simulink model "kranTest"  (R2018b)
settings: Solver=VariableStepAuto  StartTime=0.0  StopTime=Tsim  FixedStep=0.005  RelTol=1e-4
model workspace: external: MATLAB File kran_DataFile.m (data not in the file)
values from neighbouring files (symbols this model uses):
  refPointsVector = [pointThree, pointOne, pointThree, pointTwo, pointThree]    [simulate_driving.m]    (also in testDriving.m)
  Ts = 50e-3    (= 0.05)    [simulation_params.m]    (also in testDriving.m = 0.1)
undefined symbols (not defined in the file or in its folder): EvaluateTrajectory, smiData, X, Y, Z
libraries: sm_lib x105, nesl_utility x32, fl_lib x27, sh_lib x9, elec_lib x2
(part 1 of 4)
settings Model: Creator=Marko  LastModifiedBy=Marko
settings SimscapeCC: SimscapeLogType=all  SimscapeLogSimulationStatistics=on  SimscapeLogLimitData=off
settings ExplorerConfigSet: InternalSimMechanicsExplorerSettings="<ExplorerConfiguration><canonicalview>planar_xy</canonicalview><AnimationSetting><BasePlaybackSpeed>1.0</BasePlaybackSpeed><PlaybackSpeedFactor>1.0</PlaybackSpeedFactor></AnimationSetting><TilePanel><TileInfo><Tiles Columns=\"1\" Count=\"1\" Rows=\"1\"><Column Weight=\"1\"/><Row Weight=\"1\"/><Tile Height=\"1\" Width=\"1\" X=\"0\" Y=\"0\"/></Tiles></TileInfo><SceneInfo><SceneViewer><BGColor><R>0.60000002384185791</R><G>0.60000002384185791</G><B>0.60000002384185791</B></BGColor><Camera><DoPerspective>off</DoPerspective><Position><X>10.1383469879859511</X><Y>3.51643315137439361</Y><Z>-1.36564695488922516</Z></Position><Center><X>1.28157942243814538</X><Y>3.51643315137439361</Y><Z>-1.36564695488922516</Z></Center><Up><X>0</X><Y>1</Y><Z>0</Z></Up><ViewLimDist>1</ViewLimDist><YLim>6.81084416950491534</YLim><XLim>4.8510498406429976</XLim></Camera></SceneViewer></SceneInfo></TilePanel><MechEditorPanel><Cameras/><GfxPanelCameraMap/><VideoCreator><PlaybackSpeedRatio>1.0</PlaybackSpeedRatio><FrameRate>30</FrameRate><VideoFormat>Motion JPEG AVI</VideoFormat><FrameSize>auto</FrameSize></VideoCreator></MechEditorPanel></ExplorerConfiguration>"

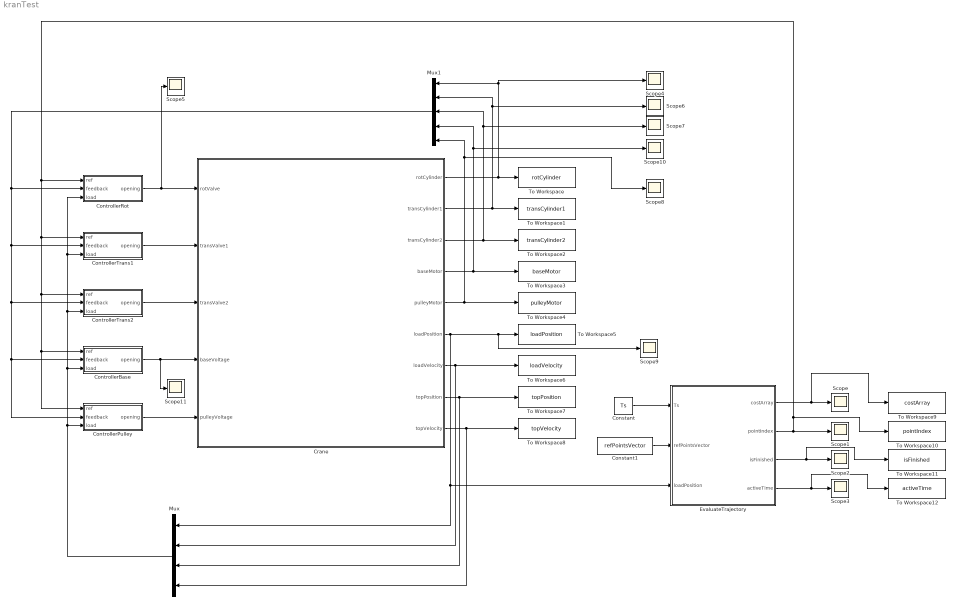
== system kranTest ==
  Constant : Constant  Value=Ts  SampleTime=-1
  Constant1 : Constant  Value=refPointsVector  SampleTime=-1
  ControllerBase : Subsystem
  ControllerPulley : Subsystem
  ControllerRot : Subsystem
  ControllerTrans1 : Subsystem
  ControllerTrans2 : Subsystem
  Crane : Subsystem
  EvaluateTrajectory : Subsystem
  Mux : Mux
  Mux1 : Mux  Inputs=5
  Scope{,1..11} (12 alike) : Scope
  To Workspace : ToWorkspace  VariableName=rotCylinder  SaveFormat=Structure With Time  SampleTime=Ts
  To Workspace1 : ToWorkspace  VariableName=transCylinder1  SaveFormat=Structure With Time  SampleTime=Ts
  To Workspace10 : ToWorkspace  VariableName=pointIndex  SaveFormat=Structure With Time  SampleTime=Ts
  To Workspace11 : ToWorkspace  VariableName=isFinished  SaveFormat=Structure With Time  SampleTime=Ts
  To Workspace12 : ToWorkspace  VariableName=activeTime  SaveFormat=Structure With Time  SampleTime=Ts
  To Workspace2 : ToWorkspace  VariableName=transCylinder2  SaveFormat=Structure With Time  SampleTime=Ts
  To Workspace3 : ToWorkspace  VariableName=baseMotor  SaveFormat=Structure With Time  SampleTime=Ts
  To Workspace4 : ToWorkspace  VariableName=pulleyMotor  SaveFormat=Structure With Time  SampleTime=Ts
  To Workspace5 : ToWorkspace  VariableName=loadPosition  SaveFormat=Structure With Time  SampleTime=Ts
  To Workspace6 : ToWorkspace  VariableName=loadVelocity  SaveFormat=Structure With Time  SampleTime=Ts
  To Workspace7 : ToWorkspace  VariableName=topPosition  SaveFormat=Structure With Time  SampleTime=Ts
  To Workspace8 : ToWorkspace  VariableName=topVelocity  SaveFormat=Structure With Time  SampleTime=Ts
  To Workspace9 : ToWorkspace  VariableName=costArray  SaveFormat=Structure With Time  SampleTime=Ts
  wires:
  Crane/1(rotCylinder) -> Scope4/1, Mux1/1, To Workspace/1
  Crane/2(transCylinder1) -> Mux1/2, Scope6/1, To Workspace1/1
  Crane/3(transCylinder2) -> Scope7/1, Mux1/3, To Workspace2/1
  Crane/4(baseMotor) -> Scope10/1, Mux1/4, To Workspace3/1
  Crane/5(pulleyMotor) -> Mux1/5, Scope8/1, To Workspace4/1
  Crane/6(loadPosition) -> Scope9/1, To Workspace5/1, EvaluateTrajectory/3(loadPosition), Mux/1
  Crane/7(loadVelocity) -> Mux/2, To Workspace6/1
  Crane/8(topPosition) -> Mux/3, To Workspace7/1
  Crane/9(topVelocity) -> Mux/4, To Workspace8/1
  Mux/1 -> ControllerRot/3(load), ControllerTrans1/3(load), ControllerTrans2/3(load), ControllerBase/3(load), ControllerPulley/3(load)
  Constant/1 -> EvaluateTrajectory/1(Ts)
  Constant1/1 -> EvaluateTrajectory/2(refPointsVector)
  EvaluateTrajectory/1(costArray) -> To Workspace9/1, Scope/1
  EvaluateTrajectory/3(isFinished) -> To Workspace11/1, Scope2/1
  EvaluateTrajectory/4(activeTime) -> To Workspace12/1, Scope3/1
  EvaluateTrajectory/2(pointIndex) -> To Workspace10/1, ControllerRot/1(ref), ControllerPulley/1(ref), ControllerBase/1(ref), ControllerTrans2/1(ref), ControllerTrans1/1(ref), Scope1/1
  Mux1/1 -> ControllerRot/2(feedback), ControllerTrans1/2(feedback), ControllerTrans2/2(feedback), ControllerPulley/2(feedback), ControllerBase/2(feedback)
  ControllerRot/1(opening) -> Scope5/1, Crane/1(rotValve)
  ControllerTrans1/1(opening) -> Crane/2(transValve1)
  ControllerTrans2/1(opening) -> Crane/3(transValve2)
  ControllerPulley/1(opening) -> Crane/5(pulleyVoltage)
  ControllerBase/1(opening) -> Scope11/1, Crane/4(baseVoltage)

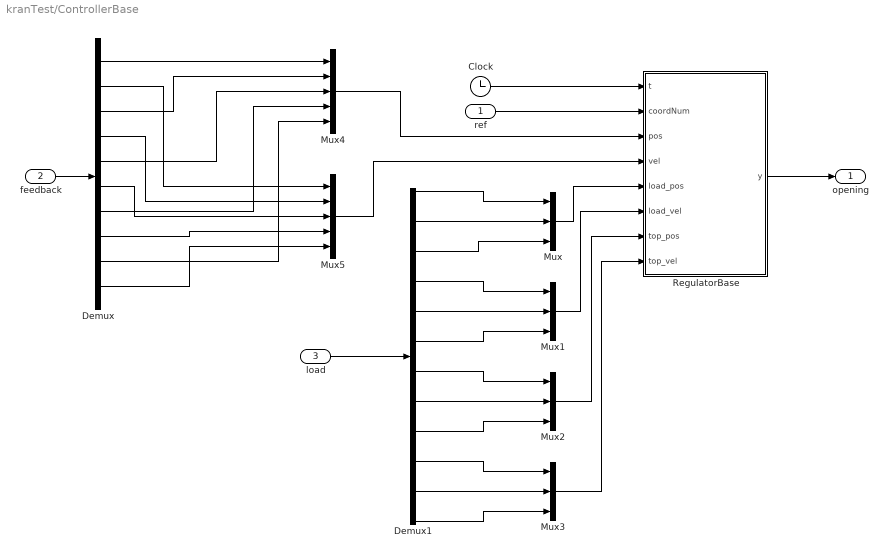
== system kranTest/ControllerBase ==
  ref : Inport
  feedback : Inport  Port=2
  load : Inport  Port=3
  Clock : Clock
  Demux : Demux  Outputs=10
  Demux1 : Demux  Outputs=12
  Mux{,1..3} (4 alike) : Mux  Inputs=3
  Mux4 : Mux  Inputs=5
  Mux5 : Mux  Inputs=5
  RegulatorBase : MATLAB Function  TreatAsAtomicUnit=on  SystemSampleTime=Ts
  opening : Outport
  wires:
  Demux1/7 -> Mux2/1
  Clock/1 -> RegulatorBase/1(t)
  Demux1/2 -> Mux/2
  Demux1/8 -> Mux2/2
  Mux1/1 -> RegulatorBase/6(load_vel)
  load/1 -> Demux1/1
  Demux1/1 -> Mux/1
  Demux1/10 -> Mux3/1
  Mux/1 -> RegulatorBase/5(load_pos)
  Mux3/1 -> RegulatorBase/8(top_vel)
  Demux1/6 -> Mux1/3
  Demux1/9 -> Mux2/3
  Mux2/1 -> RegulatorBase/7(top_pos)
  Demux1/5 -> Mux1/2
  Demux1/3 -> Mux/3
  Demux1/11 -> Mux3/2
  ref/1 -> RegulatorBase/2(coordNum)
  Demux1/12 -> Mux3/3
  RegulatorBase/1(y) -> opening/1
  Demux1/4 -> Mux1/1
  Mux4/1 -> RegulatorBase/3(pos)
  Demux/6 -> Mux5/3
  Demux/4 -> Mux5/2
  Demux/8 -> Mux5/4
  Demux/10 -> Mux5/5
  Demux/2 -> Mux5/1
  Demux/5 -> Mux4/3
  Demux/9 -> Mux4/5
  Demux/3 -> Mux4/2
  Demux/1 -> Mux4/1
  Demux/7 -> Mux4/4
  feedback/1 -> Demux/1
  Mux5/1 -> RegulatorBase/4(vel)

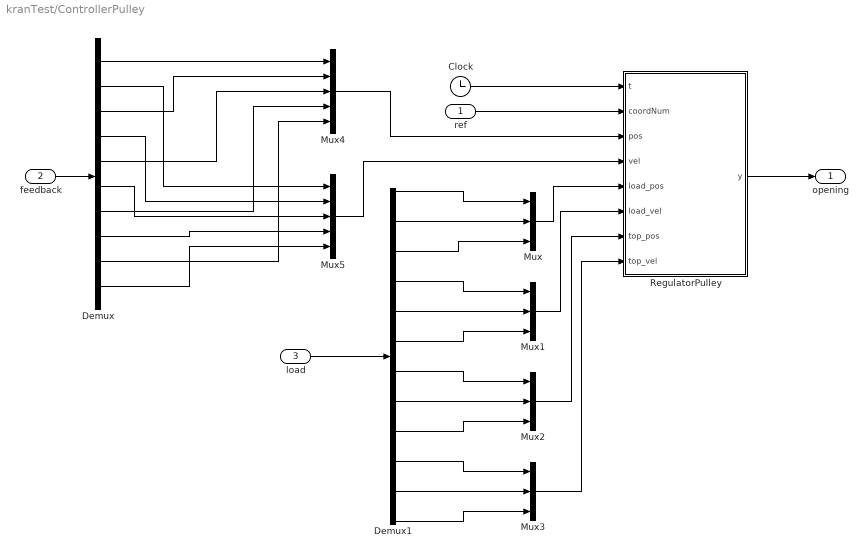
== system kranTest/ControllerPulley ==
  ref : Inport
  feedback : Inport  Port=2
  load : Inport  Port=3
  Clock : Clock
  Demux : Demux  Outputs=10
  Demux1 : Demux  Outputs=12
  Mux{,1..3} (4 alike) : Mux  Inputs=3
  Mux4 : Mux  Inputs=5
  Mux5 : Mux  Inputs=5
  RegulatorPulley : MATLAB Function  TreatAsAtomicUnit=on  SystemSampleTime=Ts
  opening : Outport
  wires:
  Demux1/7 -> Mux2/1
  Clock/1 -> RegulatorPulley/1(t)
  Demux1/2 -> Mux/2
  Demux1/8 -> Mux2/2
  Mux1/1 -> RegulatorPulley/6(load_vel)
  load/1 -> Demux1/1
  Demux1/1 -> Mux/1
  Demux1/10 -> Mux3/1
  Mux/1 -> RegulatorPulley/5(load_pos)
  Mux3/1 -> RegulatorPulley/8(top_vel)
  Demux1/6 -> Mux1/3
  Demux1/9 -> Mux2/3
  Mux2/1 -> RegulatorPulley/7(top_pos)
  Demux1/5 -> Mux1/2
  Demux1/3 -> Mux/3
  Demux1/11 -> Mux3/2
  ref/1 -> RegulatorPulley/2(coordNum)
  Demux1/12 -> Mux3/3
  RegulatorPulley/1(y) -> opening/1
  Demux1/4 -> Mux1/1
  Demux/6 -> Mux5/3
  Demux/4 -> Mux5/2
  Demux/8 -> Mux5/4
  Demux/10 -> Mux5/5
  Demux/2 -> Mux5/1
  Demux/5 -> Mux4/3
  Demux/9 -> Mux4/5
  Demux/3 -> Mux4/2
  Demux/1 -> Mux4/1
  Demux/7 -> Mux4/4
  feedback/1 -> Demux/1
  Mux4/1 -> RegulatorPulley/3(pos)
  Mux5/1 -> RegulatorPulley/4(vel)

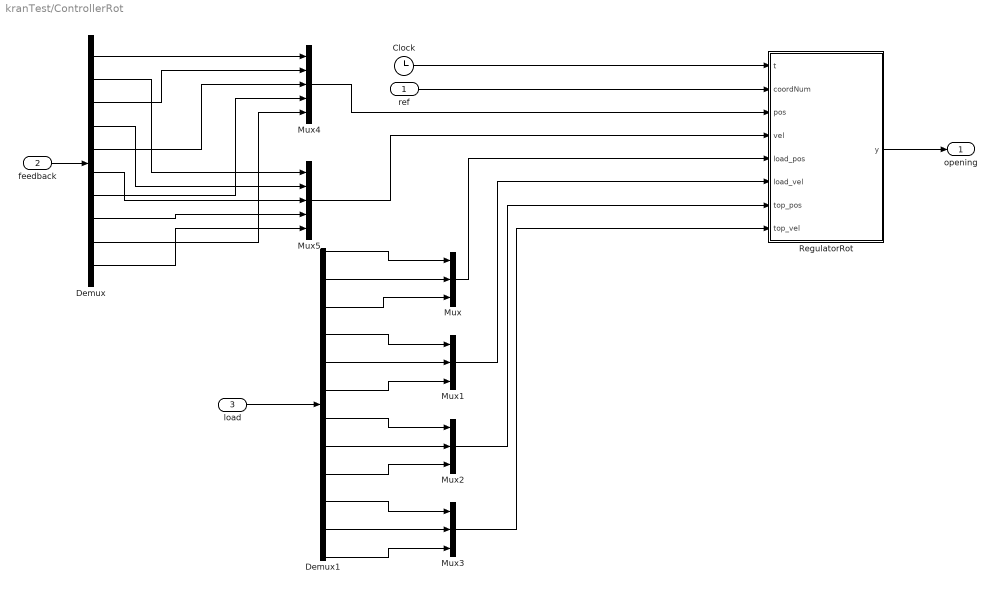
== system kranTest/ControllerRot ==
  ref : Inport
  feedback : Inport  Port=2
  load : Inport  Port=3
  Clock : Clock
  Demux : Demux  Outputs=10
  Demux1 : Demux  Outputs=12
  Mux{,1..3} (4 alike) : Mux  Inputs=3
  Mux4 : Mux  Inputs=5
  Mux5 : Mux  Inputs=5
  RegulatorRot : MATLAB Function  TreatAsAtomicUnit=on  SystemSampleTime=Ts
  opening : Outport
  wires:
  RegulatorRot/1(y) -> opening/1
  ref/1 -> RegulatorRot/2(coordNum)
  Clock/1 -> RegulatorRot/1(t)
  load/1 -> Demux1/1
  Mux/1 -> RegulatorRot/5(load_pos)
  Mux1/1 -> RegulatorRot/6(load_vel)
  Mux2/1 -> RegulatorRot/7(top_pos)
  Mux3/1 -> RegulatorRot/8(top_vel)
  Demux1/1 -> Mux/1
  Demux1/2 -> Mux/2
  Demux1/3 -> Mux/3
  Demux1/4 -> Mux1/1
  Demux1/5 -> Mux1/2
  Demux1/6 -> Mux1/3
  Demux1/7 -> Mux2/1
  Demux1/8 -> Mux2/2
  Demux1/9 -> Mux2/3
  Demux1/10 -> Mux3/1
  Demux1/11 -> Mux3/2
  Demux1/12 -> Mux3/3
  Demux/1 -> Mux4/1
  Demux/3 -> Mux4/2
  Demux/5 -> Mux4/3
  Demux/7 -> Mux4/4
  Demux/9 -> Mux4/5
  Demux/2 -> Mux5/1
  Demux/4 -> Mux5/2
  Demux/6 -> Mux5/3
  Demux/8 -> Mux5/4
  Demux/10 -> Mux5/5
  Mux4/1 -> RegulatorRot/3(pos)
  Mux5/1 -> RegulatorRot/4(vel)
  feedback/1 -> Demux/1

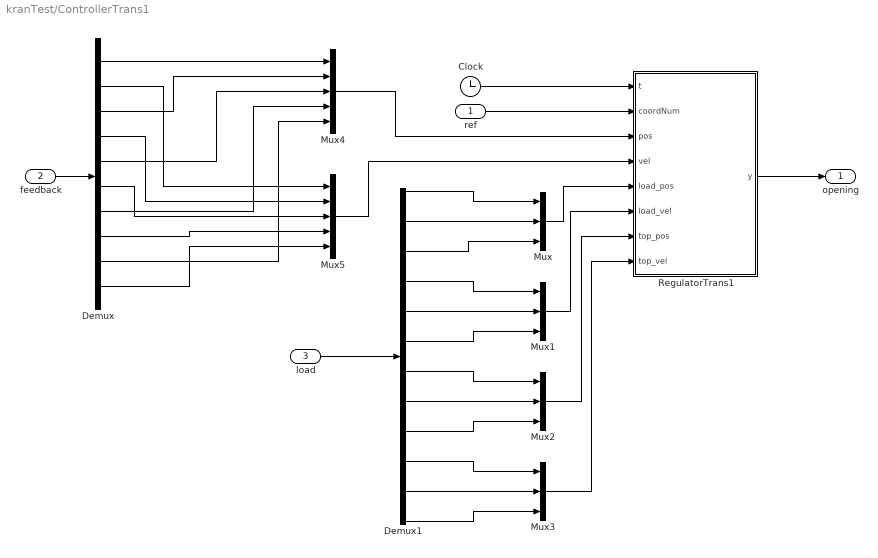
== system kranTest/ControllerTrans1 ==
  ref : Inport
  feedback : Inport  Port=2
  load : Inport  Port=3
  Clock : Clock
  Demux : Demux  Outputs=10
  Demux1 : Demux  Outputs=12
  Mux{,1..3} (4 alike) : Mux  Inputs=3
  Mux4 : Mux  Inputs=5
  Mux5 : Mux  Inputs=5
  RegulatorTrans1 : MATLAB Function  TreatAsAtomicUnit=on  SystemSampleTime=Ts
  opening : Outport
  wires:
  Demux1/7 -> Mux2/1
  Clock/1 -> RegulatorTrans1/1(t)
  Demux1/2 -> Mux/2
  Demux1/8 -> Mux2/2
  Mux1/1 -> RegulatorTrans1/6(load_vel)
  load/1 -> Demux1/1
  Demux1/1 -> Mux/1
  Demux1/10 -> Mux3/1
  Mux/1 -> RegulatorTrans1/5(load_pos)
  Mux3/1 -> RegulatorTrans1/8(top_vel)
  Demux1/6 -> Mux1/3
  Demux1/9 -> Mux2/3
  Mux2/1 -> RegulatorTrans1/7(top_pos)
  Demux1/5 -> Mux1/2
  Demux1/3 -> Mux/3
  Demux1/11 -> Mux3/2
  ref/1 -> RegulatorTrans1/2(coordNum)
  Demux1/12 -> Mux3/3
  RegulatorTrans1/1(y) -> opening/1
  Demux1/4 -> Mux1/1
  Demux/6 -> Mux5/3
  Demux/4 -> Mux5/2
  Demux/8 -> Mux5/4
  Demux/10 -> Mux5/5
  Demux/2 -> Mux5/1
  Demux/5 -> Mux4/3
  Demux/9 -> Mux4/5
  Demux/3 -> Mux4/2
  Demux/1 -> Mux4/1
  Demux/7 -> Mux4/4
  feedback/1 -> Demux/1
  Mux4/1 -> RegulatorTrans1/3(pos)
  Mux5/1 -> RegulatorTrans1/4(vel)

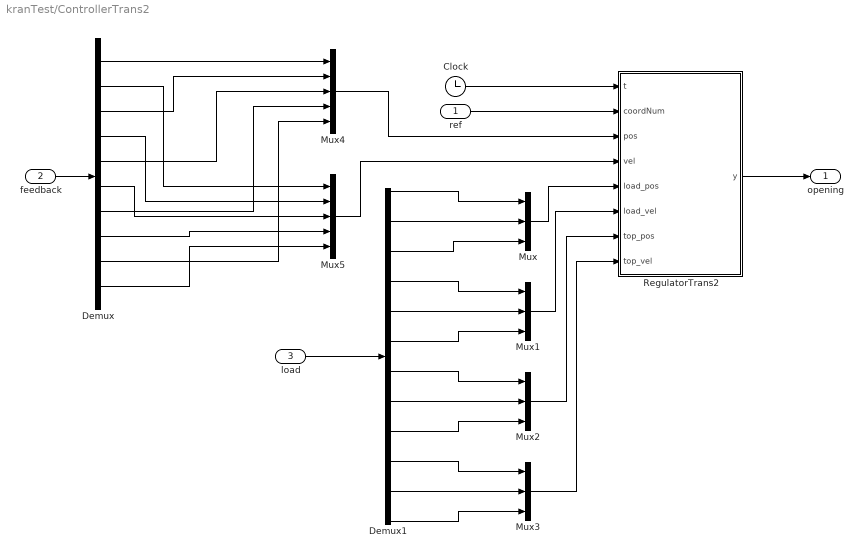
== system kranTest/ControllerTrans2 ==
  ref : Inport
  feedback : Inport  Port=2
  load : Inport  Port=3
  Clock : Clock
  Demux : Demux  Outputs=10
  Demux1 : Demux  Outputs=12
  Mux{,1..3} (4 alike) : Mux  Inputs=3
  Mux4 : Mux  Inputs=5
  Mux5 : Mux  Inputs=5
  RegulatorTrans2 : MATLAB Function  TreatAsAtomicUnit=on  SystemSampleTime=Ts
  opening : Outport
  wires:
  Demux1/7 -> Mux2/1
  Clock/1 -> RegulatorTrans2/1(t)
  Demux1/2 -> Mux/2
  Demux1/8 -> Mux2/2
  Mux1/1 -> RegulatorTrans2/6(load_vel)
  load/1 -> Demux1/1
  Demux1/1 -> Mux/1
  Demux1/10 -> Mux3/1
  Mux/1 -> RegulatorTrans2/5(load_pos)
  Mux3/1 -> RegulatorTrans2/8(top_vel)
  Demux1/6 -> Mux1/3
  Demux1/9 -> Mux2/3
  Mux2/1 -> RegulatorTrans2/7(top_pos)
  Demux1/5 -> Mux1/2
  Demux1/3 -> Mux/3
  Demux1/11 -> Mux3/2
  ref/1 -> RegulatorTrans2/2(coordNum)
  Demux1/12 -> Mux3/3
  RegulatorTrans2/1(y) -> opening/1
  Demux1/4 -> Mux1/1
  Demux/6 -> Mux5/3
  Demux/4 -> Mux5/2
  Demux/8 -> Mux5/4
  Demux/10 -> Mux5/5
  Demux/2 -> Mux5/1
  Demux/5 -> Mux4/3
  Demux/9 -> Mux4/5
  Demux/3 -> Mux4/2
  Demux/1 -> Mux4/1
  Demux/7 -> Mux4/4
  feedback/1 -> Demux/1
  Mux4/1 -> RegulatorTrans2/3(pos)
  Mux5/1 -> RegulatorTrans2/4(vel)

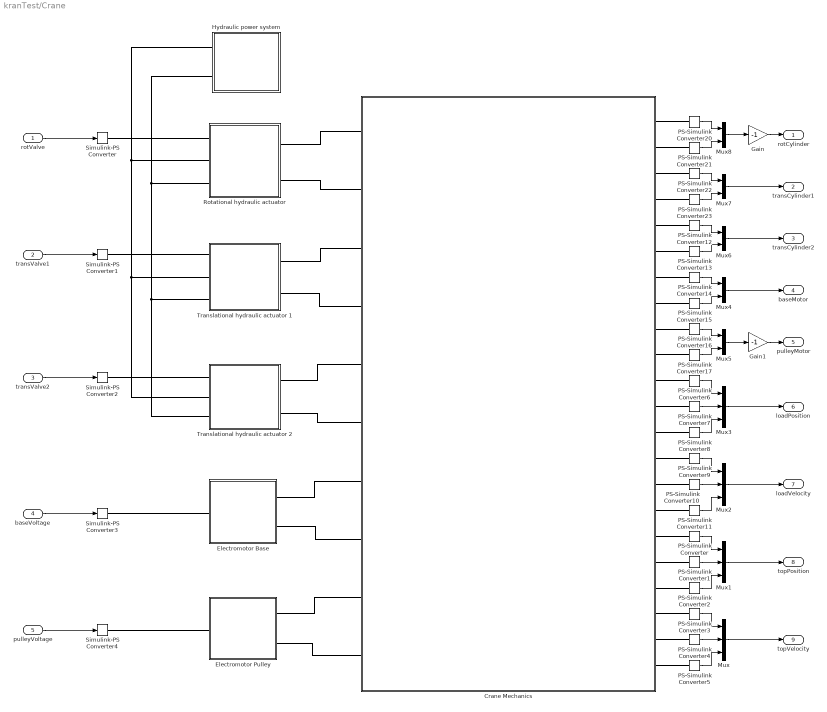
== system kranTest/Crane ==
  rotValve : Inport
  transValve1 : Inport  Port=2
  transValve2 : Inport  Port=3
  baseVoltage : Inport  Port=4
  pulleyVoltage : Inport  Port=5
  Crane Mechanics : Subsystem
  Electromotor Base : Subsystem
  Electromotor Pulley : Subsystem
  Gain : Gain  Gain=-1
  Gain1 : Gain  Gain=-1
  Hydraulic power system : Subsystem
  Mux{,1..3} (4 alike) : Mux  Inputs=3
  Mux{4..8} (5 alike) : Mux  Inputs=2
  PS-Simulink Converter{,1..17,20..23} (22 alike) : nesl_utility/PS-Simulink Converter  PhysicalDomain=network_engine_domain  SubClassName=ps_output  LeftPortType=input  RightPortType=output  PseudoPeriodic=off  Frequencies=[]  Unit=1  AffineConversion=off
  Rotational hydraulic actuator : Subsystem
  Simulink-PS Converter : nesl_utility/Simulink-PS Converter  PhysicalDomain=network_engine_domain  SubClassName=ps_input  LeftPortType=input  RightPortType=output  PseudoPeriodic=off  Frequencies=[]  NoiseDistribution=none  NoiseParameters=[]  Unit=1  AffineConversion=off  FilteringAndDerivatives=provide  SimscapeFilterOrder=1  InputFilterTimeConstant=0.001  UdotUserProvided=0
  Simulink-PS Converter{1..4} (4 alike) : nesl_utility/Simulink-PS Converter  PhysicalDomain=network_engine_domain  SubClassName=ps_input  LeftPortType=input  RightPortType=output  PseudoPeriodic=off  Frequencies=[]  NoiseDistribution=none  NoiseParameters=[]  Unit=1  AffineConversion=off  FilteringAndDerivatives=provide  SimscapeFilterOrder=2  InputFilterTimeConstant=0.001  UdotUserProvided=0
  Translational hydraulic actuator 1 : Subsystem
  Translational hydraulic actuator 2 : Subsystem
  rotCylinder : Outport
  transCylinder1 : Outport  Port=2
  transCylinder2 : Outport  Port=3
  baseMotor : Outport  Port=4
  pulleyMotor : Outport  Port=5
  loadPosition : Outport  Port=6
  loadVelocity : Outport  Port=7
  topPosition : Outport  Port=8
  topVelocity : Outport  Port=9
  wires:
  PS-Simulink Converter12/1 -> Mux6/1
  Mux2/1 -> loadVelocity/1
  PS-Simulink Converter11/1 -> Mux2/3
  PS-Simulink Converter22/1 -> Mux7/1
  Mux3/1 -> loadPosition/1
  PS-Simulink Converter4/1 -> Mux/2
  PS-Simulink Converter17/1 -> Mux5/2
  PS-Simulink Converter15/1 -> Mux4/2
  PS-Simulink Converter1/1 -> Mux1/2
  PS-Simulink Converter/1 -> Mux1/1
  PS-Simulink Converter21/1 -> Mux8/2
  PS-Simulink Converter9/1 -> Mux2/1
  PS-Simulink Converter8/1 -> Mux3/3
  PS-Simulink Converter10/1 -> Mux2/2
  PS-Simulink Converter6/1 -> Mux3/1
  PS-Simulink Converter14/1 -> Mux4/1
  PS-Simulink Converter13/1 -> Mux6/2
  Mux6/1 -> transCylinder2/1
  PS-Simulink Converter16/1 -> Mux5/1
  PS-Simulink Converter3/1 -> Mux/1
  PS-Simulink Converter20/1 -> Mux8/1
  PS-Simulink Converter23/1 -> Mux7/2
  Mux1/1 -> topPosition/1
  PS-Simulink Converter5/1 -> Mux/3
  PS-Simulink Converter2/1 -> Mux1/3
  PS-Simulink Converter7/1 -> Mux3/2
  Mux7/1 -> transCylinder1/1
  Mux4/1 -> baseMotor/1
  Mux/1 -> topVelocity/1
  Mux5/1 -> Gain1/1
  Mux8/1 -> Gain/1
  pulleyVoltage/1 -> Simulink-PS Converter4/1
  transValve1/1 -> Simulink-PS Converter1/1
  baseVoltage/1 -> Simulink-PS Converter3/1
  rotValve/1 -> Simulink-PS Converter/1
  transValve2/1 -> Simulink-PS Converter2/1
  Gain/1 -> rotCylinder/1
  Gain1/1 -> pulleyMotor/1
  connections:
  Crane Mechanics/RConn5 -- PS-Simulink Converter12/LConn1
  Hydraulic power system/RConn2 -- Rotational hydraulic actuator/LConn3 -- Translational hydraulic actuator 2/LConn3 -- Translational hydraulic actuator 1/LConn3
  Rotational hydraulic actuator/RConn2 -- Crane Mechanics/LConn2
  Crane Mechanics/RConn7 -- PS-Simulink Converter14/LConn1
  Hydraulic power system/RConn1 -- Rotational hydraulic actuator/LConn2 -- Translational hydraulic actuator 2/LConn2 -- Translational hydraulic actuator 1/LConn2
  Translational hydraulic actuator 1/RConn1 -- Crane Mechanics/LConn3
  Crane Mechanics/RConn14 -- PS-Simulink Converter9/LConn1
  Crane Mechanics/RConn6 -- PS-Simulink Converter13/LConn1
  Crane Mechanics/RConn15 -- PS-Simulink Converter10/LConn1
  Translational hydraulic actuator 2/RConn2 -- Crane Mechanics/LConn6
  Crane Mechanics/RConn9 -- PS-Simulink Converter16/LConn1
  Simulink-PS Converter4/RConn1 -- Electromotor Pulley/LConn1
  Electromotor Pulley/RConn2 -- Crane Mechanics/LConn10
  PS-Simulink Converter2/LConn1 -- Crane Mechanics/RConn19
  Crane Mechanics/RConn16 -- PS-Simulink Converter11/LConn1
  Crane Mechanics/RConn11 -- PS-Simulink Converter6/LConn1
  PS-Simulink Converter5/LConn1 -- Crane Mechanics/RConn22
  Rotational hydraulic actuator/RConn1 -- Crane Mechanics/LConn1
  Crane Mechanics/RConn4 -- PS-Simulink Converter23/LConn1
  Crane Mechanics/RConn13 -- PS-Simulink Converter8/LConn1
  Electromotor Base/RConn2 -- Crane Mechanics/LConn8
  Translational hydraulic actuator 1/RConn2 -- Crane Mechanics/LConn4
  PS-Simulink Converter/LConn1 -- Crane Mechanics/RConn17
  Crane Mechanics/RConn3 -- PS-Simulink Converter22/LConn1
  Crane Mechanics/LConn9 -- Electromotor Pulley/RConn1
  Crane Mechanics/RConn8 -- PS-Simulink Converter15/LConn1
  PS-Simulink Converter4/LConn1 -- Crane Mechanics/RConn21
  Crane Mechanics/RConn2 -- PS-Simulink Converter21/LConn1
  Crane Mechanics/LConn5 -- Translational hydraulic actuator 2/RConn1
  Simulink-PS Converter/RConn1 -- Rotational hydraulic actuator/LConn1
  Simulink-PS Converter3/RConn1 -- Electromotor Base/LConn1
  Simulink-PS Converter1/RConn1 -- Translational hydraulic actuator 1/LConn1
  Crane Mechanics/RConn12 -- PS-Simulink Converter7/LConn1
  Crane Mechanics/RConn1 -- PS-Simulink Converter20/LConn1
  Simulink-PS Converter2/RConn1 -- Translational hydraulic actuator 2/LConn1
  PS-Simulink Converter1/LConn1 -- Crane Mechanics/RConn18
  Crane Mechanics/LConn7 -- Electromotor Base/RConn1
  Crane Mechanics/RConn10 -- PS-Simulink Converter17/LConn1
  PS-Simulink Converter3/LConn1 -- Crane Mechanics/RConn20

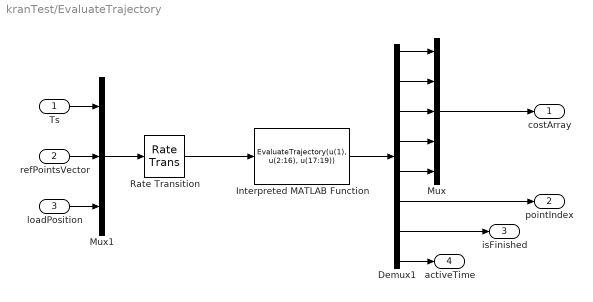
== system kranTest/EvaluateTrajectory ==
  Ts : Inport
  refPointsVector : Inport  Port=2
  loadPosition : Inport  Port=3
  Demux1 : Demux  Outputs=8
  Interpreted MATLAB Function : MATLABFcn  MATLABFcn=EvaluateTrajectory(u(1), u(2:16), u(17:19))  OutputDimensions=8  OutputSignalType=real
  Mux : Mux  Inputs=5
  Mux1 : Mux  Inputs=3
  Rate Transition : RateTransition  OutPortSampleTime=Ts
  costArray : Outport
  pointIndex : Outport  Port=2
  isFinished : Outport  Port=3
  activeTime : Outport  Port=4
  wires:
  Interpreted MATLAB Function/1 -> Demux1/1
  Rate Transition/1 -> Interpreted MATLAB Function/1
  Mux1/1 -> Rate Transition/1
  refPointsVector/1 -> Mux1/2
  Ts/1 -> Mux1/1
  loadPosition/1 -> Mux1/3
  Mux/1 -> costArray/1
  Demux1/1 -> Mux/1
  Demux1/2 -> Mux/2
  Demux1/3 -> Mux/3
  Demux1/4 -> Mux/4
  Demux1/5 -> Mux/5
  Demux1/6 -> pointIndex/1
  Demux1/7 -> isFinished/1
  Demux1/8 -> activeTime/1

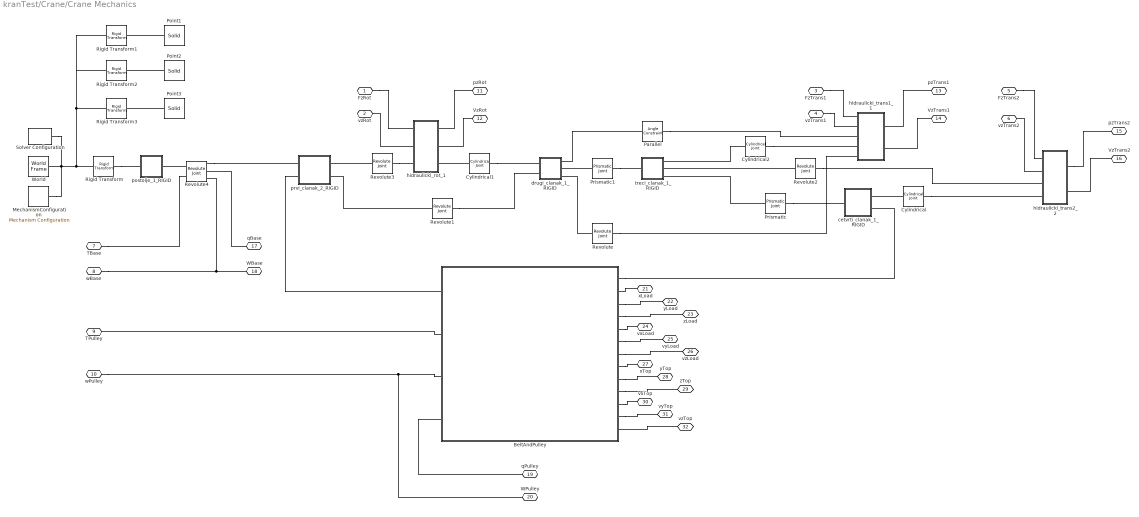
== system kranTest/Crane/Crane Mechanics ==
  BeltAndPulley : Subsystem
  Cylindrical : sm_lib/Joints/Cylindrical Joint  SenseConstraintForce=off  SenseConstraintForceX=off  SenseConstraintForceY=off  SenseConstraintForceZ=off  SenseConstraintTorque=off  SenseConstraintTorqueX=off  SenseConstraintTorqueY=off  SenseConstraintTorqueZ=off  SenseTotalForce=off  SenseTotalForceX=off  SenseTotalForceY=off  SenseTotalForceZ=off  SenseTotalTorque=off  SenseTotalTorqueX=off  SenseTotalTorqueY=off  SenseTotalTorqueZ=off  CompositeWrenchDir=FollowerOnBase  CompositeWrenchFrame=BaseFrame  PzEquilibriumPosition=0  PzEquilibriumPositionUnits=m  PzSpringStiffness=0  PzSpringStiffnessUnits=N/m  PzDampingCoefficient=0  PzDampingCoefficientUnits=N/(m/s)  PzTorqueActuationMode=NoTorque  PzMotionActuationMode=ComputedMotion  PzSensePosition=off  PzSenseVelocity=off  PzSenseAcceleration=off  PzSenseTorqueForce=off  PzPositionTargetSpecify=off  PzPositionTargetPriority=High  PzPositionTargetValue=0  PzPositionTargetValueUnits=m  PzVelocityTargetSpecify=off  PzVelocityTargetPriority=High  PzVelocityTargetValue=0  PzVelocityTargetValueUnits=m/s  RzEquilibriumPosition=0  RzEquilibriumPositionUnits=rad  RzSpringStiffness=0  RzSpringStiffnessUnits=N*m/rad  RzDampingCoefficient=0  RzDampingCoefficientUnits=N*m/(rad/s)  RzTorqueActuationMode=NoTorque  RzMotionActuationMode=ComputedMotion  RzSensePosition=off  RzSenseVelocity=off  RzSenseAcceleration=off  RzSenseTorqueForce=off  RzPositionTargetSpecify=off  RzPositionTargetPriority=High  RzPositionTargetValue=0  RzPositionTargetValueUnits=deg  RzVelocityTargetSpecify=off  RzVelocityTargetPriority=High  RzVelocityTargetValue=0  RzVelocityTargetValueUnits=deg/s
  Cylindrical1 : sm_lib/Joints/Cylindrical Joint  SenseConstraintForce=off  SenseConstraintForceX=off  SenseConstraintForceY=off  SenseConstraintForceZ=off  SenseConstraintTorque=off  SenseConstraintTorqueX=off  SenseConstraintTorqueY=off  SenseConstraintTorqueZ=off  SenseTotalForce=off  SenseTotalForceX=off  SenseTotalForceY=off  SenseTotalForceZ=off  SenseTotalTorque=off  SenseTotalTorqueX=off  SenseTotalTorqueY=off  SenseTotalTorqueZ=off  CompositeWrenchDir=FollowerOnBase  CompositeWrenchFrame=BaseFrame  PzEquilibriumPosition=0  PzEquilibriumPositionUnits=m  PzSpringStiffness=0  PzSpringStiffnessUnits=N/m  PzDampingCoefficient=0  PzDampingCoefficientUnits=N/(m/s)  PzTorqueActuationMode=NoTorque  PzMotionActuationMode=ComputedMotion  PzSensePosition=off  PzSenseVelocity=off  PzSenseAcceleration=off  PzSenseTorqueForce=off  PzPositionTargetSpecify=off  PzPositionTargetPriority=High  PzPositionTargetValue=0  PzPositionTargetValueUnits=m  PzVelocityTargetSpecify=off  PzVelocityTargetPriority=High  PzVelocityTargetValue=0  PzVelocityTargetValueUnits=m/s  RzEquilibriumPosition=0  RzEquilibriumPositionUnits=rad  RzSpringStiffness=0  RzSpringStiffnessUnits=N*m/rad  RzDampingCoefficient=0  RzDampingCoefficientUnits=N*m/(rad/s)  RzTorqueActuationMode=NoTorque  RzMotionActuationMode=ComputedMotion  RzSensePosition=off  RzSenseVelocity=off  RzSenseAcceleration=off  RzSenseTorqueForce=off  RzPositionTargetSpecify=off  RzPositionTargetPriority=High  RzPositionTargetValue=0  RzPositionTargetValueUnits=deg  RzVelocityTargetSpecify=off  RzVelocityTargetPriority=High  RzVelocityTargetValue=0  RzVelocityTargetValueUnits=deg/s
  Cylindrical2 : sm_lib/Joints/Cylindrical Joint  SenseConstraintForce=off  SenseConstraintForceX=off  SenseConstraintForceY=off  SenseConstraintForceZ=off  SenseConstraintTorque=off  SenseConstraintTorqueX=off  SenseConstraintTorqueY=off  SenseConstraintTorqueZ=off  SenseTotalForce=off  SenseTotalForceX=off  SenseTotalForceY=off  SenseTotalForceZ=off  SenseTotalTorque=off  SenseTotalTorqueX=off  SenseTotalTorqueY=off  SenseTotalTorqueZ=off  CompositeWrenchDir=FollowerOnBase  CompositeWrenchFrame=BaseFrame  PzEquilibriumPosition=0  PzEquilibriumPositionUnits=m  PzSpringStiffness=0  PzSpringStiffnessUnits=N/m  PzDampingCoefficient=0  PzDampingCoefficientUnits=N/(m/s)  PzTorqueActuationMode=NoTorque  PzMotionActuationMode=ComputedMotion  PzSensePosition=off  PzSenseVelocity=off  PzSenseAcceleration=off  PzSenseTorqueForce=off  PzPositionTargetSpecify=off  PzPositionTargetPriority=High  PzPositionTargetValue=0  PzPositionTargetValueUnits=m  PzVelocityTargetSpecify=off  PzVelocityTargetPriority=High  PzVelocityTargetValue=0  PzVelocityTargetValueUnits=m/s  RzEquilibriumPosition=0  RzEquilibriumPositionUnits=rad  RzSpringStiffness=0  RzSpringStiffnessUnits=N*m/rad  RzDampingCoefficient=0  RzDampingCoefficientUnits=N*m/(rad/s)  RzTorqueActuationMode=NoTorque  RzMotionActuationMode=ComputedMotion  RzSensePosition=off  RzSenseVelocity=off  RzSenseAcceleration=off  RzSenseTorqueForce=off  RzPositionTargetSpecify=off  RzPositionTargetPriority=High  RzPositionTargetValue=0  RzPositionTargetValueUnits=deg  RzVelocityTargetSpecify=off  RzVelocityTargetPriority=High  RzVelocityTargetValue=0  RzVelocityTargetValueUnits=deg/s
  MechanismConfiguration : sm_lib/Utilities/Mechanism Configuration  UniformGravity=Constant  GravityVector=[0 -9.80665 0]  GravityUnits=m/s^2  LinearizationDelta=0.001
  Parallel : sm_lib/Constraints/Angle Constraint  ConstraintType=Parallel  Angle=45  AngleUnits=deg  SenseSignedTorqueMagnitude=off  SenseTorque=off  SenseForce=off  WrenchDir=FollowerOnBase  WrenchFrame=BaseFrame
      settings: SourceProductName=Simscape Multibody  SourceProductBaseCode=MS
  Point1 : sm_lib/Body Elements/Solid  InertiaType=CalculateFromGeometry  Mass=1  MassUnits=kg  CenterOfMass=[0 0 0]  CenterOfMassUnits=m  MomentsOfInertia=[1 1 1]  MomentsOfInertiaUnits=kg*m^2  ProductsOfInertia=[0 0 0]  ProductsOfInertiaUnits=kg*m^2  BasedOnType=Density  Density=1000  DensityUnits=kg/m^3  DoExposeReferenceFrame=on  SerializedFrames=<Frames/>  GraphicType=FromGeometry  MarkerShape=Sphere  MarkerSize=10  GraphicVisPropType=AdvancedVisualProperties  GraphicDiffuseColor=[0 1 0]  GraphicSpecularColor=[0.5 0.5 0.5 1.0]  GraphicAmbientColor=[0.15 0.15 0.15 1.0]  GraphicEmissiveColor=[0.0 0.0 0.0 1.0]  GraphicShininess=75  GraphicOpacity=1.0  GeometryShape=Sphere  RectangleSize=[1 1]  RectangleSizeUnits=m  BrickDimensions=[1 1 1]  BrickDimensionUnits=m  CylinderRadius=1  CylinderRadiusUnits=m  CylinderLength=1  CylinderLengthUnits=m  SphereRadius=0.25  SphereRadiusUnits=m  EllipsoidRadii=[1 1 1]  EllipsoidRadiiUnits=m  ExtrusionCrossSection=[1 1; -1 1; -1 -1; 1 -1]  ExtrusionCrossSectionUnits=m  ExtrusionLength=1  ExtrusionLengthUnits=m  PolygonNumSides=3  PolygonOuterRadius=1  PolygonOuterRadiusUnits=m  ExtGeomFileType=STEP  ExtGeomFileUnits=m  RevolutionCrossSection=[1 1; 1 -1; 2 -1; 2 1]  RevolutionCrossSectionUnits=m  RevolutionExtent=Full  RevolutionAngle=180  RevolutionAngleUnits=deg
  Point2 : sm_lib/Body Elements/Solid  InertiaType=CalculateFromGeometry  Mass=1  MassUnits=kg  CenterOfMass=[0 0 0]  CenterOfMassUnits=m  MomentsOfInertia=[1 1 1]  MomentsOfInertiaUnits=kg*m^2  ProductsOfInertia=[0 0 0]  ProductsOfInertiaUnits=kg*m^2  BasedOnType=Density  Density=1000  DensityUnits=kg/m^3  DoExposeReferenceFrame=on  SerializedFrames=<Frames/>  GraphicType=FromGeometry  MarkerShape=Sphere  MarkerSize=10  GraphicVisPropType=AdvancedVisualProperties  GraphicDiffuseColor=[0 0 1]  GraphicSpecularColor=[0.5 0.5 0.5 1.0]  GraphicAmbientColor=[0.15 0.15 0.15 1.0]  GraphicEmissiveColor=[0.0 0.0 0.0 1.0]  GraphicShininess=75  GraphicOpacity=1.0  GeometryShape=Sphere  RectangleSize=[1 1]  RectangleSizeUnits=m  BrickDimensions=[1 1 1]  BrickDimensionUnits=m  CylinderRadius=1  CylinderRadiusUnits=m  CylinderLength=1  CylinderLengthUnits=m  SphereRadius=0.25  SphereRadiusUnits=m  EllipsoidRadii=[1 1 1]  EllipsoidRadiiUnits=m  ExtrusionCrossSection=[1 1; -1 1; -1 -1; 1 -1]  ExtrusionCrossSectionUnits=m  ExtrusionLength=1  ExtrusionLengthUnits=m  PolygonNumSides=3  PolygonOuterRadius=1  PolygonOuterRadiusUnits=m  ExtGeomFileType=STEP  ExtGeomFileUnits=m  RevolutionCrossSection=[1 1; 1 -1; 2 -1; 2 1]  RevolutionCrossSectionUnits=m  RevolutionExtent=Full  RevolutionAngle=180  RevolutionAngleUnits=deg
  Point3 : sm_lib/Body Elements/Solid  InertiaType=CalculateFromGeometry  Mass=1  MassUnits=kg  CenterOfMass=[0 0 0]  CenterOfMassUnits=m  MomentsOfInertia=[1 1 1]  MomentsOfInertiaUnits=kg*m^2  ProductsOfInertia=[0 0 0]  ProductsOfInertiaUnits=kg*m^2  BasedOnType=Density  Density=1000  DensityUnits=kg/m^3  DoExposeReferenceFrame=on  SerializedFrames=<Frames/>  GraphicType=FromGeometry  MarkerShape=Sphere  MarkerSize=10  GraphicVisPropType=AdvancedVisualProperties  GraphicDiffuseColor=[1 0 0]  GraphicSpecularColor=[0.5 0.5 0.5 1.0]  GraphicAmbientColor=[0.15 0.15 0.15 1.0]  GraphicEmissiveColor=[0.0 0.0 0.0 1.0]  GraphicShininess=75  GraphicOpacity=1.0  GeometryShape=Sphere  RectangleSize=[1 1]  RectangleSizeUnits=m  BrickDimensions=[1 1 1]  BrickDimensionUnits=m  CylinderRadius=1  CylinderRadiusUnits=m  CylinderLength=1  CylinderLengthUnits=m  SphereRadius=0.25  SphereRadiusUnits=m  EllipsoidRadii=[1 1 1]  EllipsoidRadiiUnits=m  ExtrusionCrossSection=[1 1; -1 1; -1 -1; 1 -1]  ExtrusionCrossSectionUnits=m  ExtrusionLength=1  ExtrusionLengthUnits=m  PolygonNumSides=3  PolygonOuterRadius=1  PolygonOuterRadiusUnits=m  ExtGeomFileType=STEP  ExtGeomFileUnits=m  RevolutionCrossSection=[1 1; 1 -1; 2 -1; 2 1]  RevolutionCrossSectionUnits=m  RevolutionExtent=Full  RevolutionAngle=180  RevolutionAngleUnits=deg
  Prismatic : sm_lib/Joints/Prismatic Joint  SenseConstraintForce=off  SenseConstraintForceX=off  SenseConstraintForceY=off  SenseConstraintForceZ=off  SenseConstraintTorque=off  SenseConstraintTorqueX=off  SenseConstraintTorqueY=off  SenseConstraintTorqueZ=off  SenseTotalForce=off  SenseTotalForceX=off  SenseTotalForceY=off  SenseTotalForceZ=off  SenseTotalTorque=off  SenseTotalTorqueX=off  SenseTotalTorqueY=off  SenseTotalTorqueZ=off  CompositeWrenchDir=FollowerOnBase  CompositeWrenchFrame=BaseFrame  EquilibriumPosition=0  EquilibriumPositionUnits=m  SpringStiffness=0  SpringStiffnessUnits=N/m  DampingCoefficient=0  DampingCoefficientUnits=N/(m/s)  TorqueActuationMode=NoTorque  MotionActuationMode=ComputedMotion  SensePosition=off  SenseVelocity=off  SenseAcceleration=off  SenseTorqueForce=off  PositionTargetSpecify=on  PositionTargetPriority=Low  PositionTargetValue=smiData.PrismaticJoint(1).Pz.Pos  PositionTargetValueUnits=m  VelocityTargetSpecify=off  VelocityTargetPriority=High  VelocityTargetValue=0  VelocityTargetValueUnits=m/s
  Prismatic1 : sm_lib/Joints/Prismatic Joint  SenseConstraintForce=off  SenseConstraintForceX=off  SenseConstraintForceY=off  SenseConstraintForceZ=off  SenseConstraintTorque=off  SenseConstraintTorqueX=off  SenseConstraintTorqueY=off  SenseConstraintTorqueZ=off  SenseTotalForce=off  SenseTotalForceX=off  SenseTotalForceY=off  SenseTotalForceZ=off  SenseTotalTorque=off  SenseTotalTorqueX=off  SenseTotalTorqueY=off  SenseTotalTorqueZ=off  CompositeWrenchDir=FollowerOnBase  CompositeWrenchFrame=BaseFrame  EquilibriumPosition=0  EquilibriumPositionUnits=m  SpringStiffness=0  SpringStiffnessUnits=N/m  DampingCoefficient=0  DampingCoefficientUnits=N/(m/s)  TorqueActuationMode=NoTorque  MotionActuationMode=ComputedMotion  SensePosition=off  SenseVelocity=off  SenseAcceleration=off  SenseTorqueForce=off  PositionTargetSpecify=on  PositionTargetPriority=Low  PositionTargetValue=smiData.PrismaticJoint(2).Pz.Pos  PositionTargetValueUnits=m  VelocityTargetSpecify=off  VelocityTargetPriority=High  VelocityTargetValue=0  VelocityTargetValueUnits=m/s
  Revolute : sm_lib/Joints/Revolute Joint  SenseConstraintForce=off  SenseConstraintForceX=off  SenseConstraintForceY=off  SenseConstraintForceZ=off  SenseConstraintTorque=off  SenseConstraintTorqueX=off  SenseConstraintTorqueY=off  SenseConstraintTorqueZ=off  SenseTotalForce=off  SenseTotalForceX=off  SenseTotalForceY=off  SenseTotalForceZ=off  SenseTotalTorque=off  SenseTotalTorqueX=off  SenseTotalTorqueY=off  SenseTotalTorqueZ=off  CompositeWrenchDir=FollowerOnBase  CompositeWrenchFrame=BaseFrame  EquilibriumPosition=0  EquilibriumPositionUnits=rad  SpringStiffness=0  SpringStiffnessUnits=N*m/rad  DampingCoefficient=0  DampingCoefficientUnits=N*m/(rad/s)  TorqueActuationMode=NoTorque  MotionActuationMode=ComputedMotion  SensePosition=off  SenseVelocity=off  SenseAcceleration=off  SenseTorqueForce=off  PositionTargetSpecify=on  PositionTargetPriority=Low  PositionTargetValue=smiData.RevoluteJoint(4).Rz.Pos  PositionTargetValueUnits=deg  VelocityTargetSpecify=off  VelocityTargetPriority=High  VelocityTargetValue=0  VelocityTargetValueUnits=deg/s
  Revolute1 : sm_lib/Joints/Revolute Joint  SenseConstraintForce=off  SenseConstraintForceX=off  SenseConstraintForceY=off  SenseConstraintForceZ=off  SenseConstraintTorque=off  SenseConstraintTorqueX=off  SenseConstraintTorqueY=off  SenseConstraintTorqueZ=off  SenseTotalForce=off  SenseTotalForceX=off  SenseTotalForceY=off  SenseTotalForceZ=off  SenseTotalTorque=off  SenseTotalTorqueX=off  SenseTotalTorqueY=off  SenseTotalTorqueZ=off  CompositeWrenchDir=FollowerOnBase  CompositeWrenchFrame=BaseFrame  EquilibriumPosition=0  EquilibriumPositionUnits=rad  SpringStiffness=0  SpringStiffnessUnits=N*m/rad  DampingCoefficient=0  DampingCoefficientUnits=N*m/(rad/s)  TorqueActuationMode=NoTorque  MotionActuationMode=ComputedMotion  SensePosition=off  SenseVelocity=off  SenseAcceleration=off  SenseTorqueForce=off  PositionTargetSpecify=on  PositionTargetPriority=Low  PositionTargetValue=smiData.RevoluteJoint(5).Rz.Pos  PositionTargetValueUnits=deg  VelocityTargetSpecify=off  VelocityTargetPriority=High  VelocityTargetValue=0  VelocityTargetValueUnits=deg/s
  Revolute2 : sm_lib/Joints/Revolute Joint  SenseConstraintForce=off  SenseConstraintForceX=off  SenseConstraintForceY=off  SenseConstraintForceZ=off  SenseConstraintTorque=off  SenseConstraintTorqueX=off  SenseConstraintTorqueY=off  SenseConstraintTorqueZ=off  SenseTotalForce=off  SenseTotalForceX=off  SenseTotalForceY=off  SenseTotalForceZ=off  SenseTotalTorque=off  SenseTotalTorqueX=off  SenseTotalTorqueY=off  SenseTotalTorqueZ=off  CompositeWrenchDir=FollowerOnBase  CompositeWrenchFrame=BaseFrame  EquilibriumPosition=0  EquilibriumPositionUnits=rad  SpringStiffness=0  SpringStiffnessUnits=N*m/rad  DampingCoefficient=0  DampingCoefficientUnits=N*m/(rad/s)  TorqueActuationMode=NoTorque  MotionActuationMode=ComputedMotion  SensePosition=off  SenseVelocity=off  SenseAcceleration=off  SenseTorqueForce=off  PositionTargetSpecify=on  PositionTargetPriority=Low  PositionTargetValue=smiData.RevoluteJoint(6).Rz.Pos  PositionTargetValueUnits=deg  VelocityTargetSpecify=off  VelocityTargetPriority=High  VelocityTargetValue=0  VelocityTargetValueUnits=deg/s
  Revolute3 : sm_lib/Joints/Revolute Joint  SenseConstraintForce=off  SenseConstraintForceX=off  SenseConstraintForceY=off  SenseConstraintForceZ=off  SenseConstraintTorque=off  SenseConstraintTorqueX=off  SenseConstraintTorqueY=off  SenseConstraintTorqueZ=off  SenseTotalForce=off  SenseTotalForceX=off  SenseTotalForceY=off  SenseTotalForceZ=off  SenseTotalTorque=off  SenseTotalTorqueX=off  SenseTotalTorqueY=off  SenseTotalTorqueZ=off  CompositeWrenchDir=FollowerOnBase  CompositeWrenchFrame=BaseFrame  EquilibriumPosition=0  EquilibriumPositionUnits=rad  SpringStiffness=0  SpringStiffnessUnits=N*m/rad  DampingCoefficient=0  DampingCoefficientUnits=N*m/(rad/s)  TorqueActuationMode=NoTorque  MotionActuationMode=ComputedMotion  SensePosition=off  SenseVelocity=off  SenseAcceleration=off  SenseTorqueForce=off  PositionTargetSpecify=on  PositionTargetPriority=Low  PositionTargetValue=smiData.RevoluteJoint(7).Rz.Pos  PositionTargetValueUnits=deg  VelocityTargetSpecify=off  VelocityTargetPriority=High  VelocityTargetValue=0  VelocityTargetValueUnits=deg/s
  Revolute4 : sm_lib/Joints/Revolute Joint  SenseConstraintForce=off  SenseConstraintForceX=off  SenseConstraintForceY=off  SenseConstraintForceZ=off  SenseConstraintTorque=off  SenseConstraintTorqueX=off  SenseConstraintTorqueY=off  SenseConstraintTorqueZ=off  SenseTotalForce=off  SenseTotalForceX=off  SenseTotalForceY=off  SenseTotalForceZ=off  SenseTotalTorque=off  SenseTotalTorqueX=off  SenseTotalTorqueY=off  SenseTotalTorqueZ=off  CompositeWrenchDir=FollowerOnBase  CompositeWrenchFrame=BaseFrame  EquilibriumPosition=0  EquilibriumPositionUnits=rad  SpringStiffness=0  SpringStiffnessUnits=N*m/rad  DampingCoefficient=500  DampingCoefficientUnits=N*m/(rad/s)  TorqueActuationMode=InputTorque  MotionActuationMode=ComputedMotion  SensePosition=on  SenseVelocity=on  SenseAcceleration=off  SenseTorqueForce=off  PositionTargetSpecify=on  PositionTargetPriority=High  PositionTargetValue=smiData.RevoluteJoint(8).Rz.Pos  PositionTargetValueUnits=deg  VelocityTargetSpecify=off  VelocityTargetPriority=High  VelocityTargetValue=0  VelocityTargetValueUnits=deg/s
  Rigid Transform : sm_lib/Frames and Transforms/Rigid Transform  TranslationMethod=StandardAxis  TranslationStandardOffset=0.86  TranslationLengthUnit=m  TranslationStandardAxis=+Y  TranslationCartesianOffset=[0 0 0]  TranslationROffset=0  TranslationROffsetUnits=m  TranslationZOffset=0  TranslationZOffsetUnits=m  TranslationThetaOffset=0  TranslationThetaOffsetUnits=deg  RotationMethod=StandardAxis  RotationAngleUnits=deg  RotationStandardAxis=-Y  RotationAngle=90  RotationArbitraryAxis=[0 0 1]  FollAlignAxisA=+X  BaseAlignAxisA=+Y  FollAlignAxisB=+Y  BaseAlignAxisB=+Z  RotationSequenceAxes=FollowerAxes  RotationSequence=XYX  RotationSequenceAngles=[0 0 0]  RotationSequenceAnglesUnits=deg  RotationMatrix=[1 0 0; 0 1 0; 0 0 1]
  Rigid Transform1 : sm_lib/Frames and Transforms/Rigid Transform  TranslationMethod=Cartesian  TranslationStandardOffset=0.86  TranslationLengthUnit=m  TranslationStandardAxis=+Y  TranslationCartesianOffset=[8 5.65 0]  TranslationROffset=0  TranslationROffsetUnits=m  TranslationZOffset=0  TranslationZOffsetUnits=m  TranslationThetaOffset=0  TranslationThetaOffsetUnits=deg  RotationMethod=None  RotationAngleUnits=deg  RotationStandardAxis=-Y  RotationAngle=90  RotationArbitraryAxis=[0 0 1]  FollAlignAxisA=+X  BaseAlignAxisA=+Y  FollAlignAxisB=+Y  BaseAlignAxisB=+Z  RotationSequenceAxes=FollowerAxes  RotationSequence=XYX  RotationSequenceAngles=[0 0 0]  RotationSequenceAnglesUnits=deg  RotationMatrix=[1 0 0; 0 1 0; 0 0 1]
  Rigid Transform2 : sm_lib/Frames and Transforms/Rigid Transform  TranslationMethod=Cartesian  TranslationStandardOffset=0.86  TranslationLengthUnit=m  TranslationStandardAxis=+Y  TranslationCartesianOffset=[-7.5 3.4 7.5]  TranslationROffset=0  TranslationROffsetUnits=m  TranslationZOffset=0  TranslationZOffsetUnits=m  TranslationThetaOffset=0  TranslationThetaOffsetUnits=deg  RotationMethod=None  RotationAngleUnits=deg  RotationStandardAxis=-Y  RotationAngle=90  RotationArbitraryAxis=[0 0 1]  FollAlignAxisA=+X  BaseAlignAxisA=+Y  FollAlignAxisB=+Y  BaseAlignAxisB=+Z  RotationSequenceAxes=FollowerAxes  RotationSequence=XYX  RotationSequenceAngles=[0 0 0]  RotationSequenceAnglesUnits=deg  RotationMatrix=[1 0 0; 0 1 0; 0 0 1]
  Rigid Transform3 : sm_lib/Frames and Transforms/Rigid Transform  TranslationMethod=Cartesian  TranslationStandardOffset=0.86  TranslationLengthUnit=m  TranslationStandardAxis=+Y  TranslationCartesianOffset=[0 2.9 2.5]  TranslationROffset=0  TranslationROffsetUnits=m  TranslationZOffset=0  TranslationZOffsetUnits=m  TranslationThetaOffset=0  TranslationThetaOffsetUnits=deg  RotationMethod=None  RotationAngleUnits=deg  RotationStandardAxis=-Y  RotationAngle=90  RotationArbitraryAxis=[0 0 1]  FollAlignAxisA=+X  BaseAlignAxisA=+Y  FollAlignAxisB=+Y  BaseAlignAxisB=+Z  RotationSequenceAxes=FollowerAxes  RotationSequence=XYX  RotationSequenceAngles=[0 0 0]  RotationSequenceAnglesUnits=deg  RotationMatrix=[1 0 0; 0 1 0; 0 0 1]
  Solver Configuration : nesl_utility/Solver Configuration  PhysicalDomain=network_engine_domain  SubClassName=solver  LeftPortType=input  RightPortType=generic  Tones=[]  Harmonics=[]  SimulateNoise=off  Profile=off  UseLocalSampling=off  EnableSwitchedLinearOptims=on  FrequencyDomain=off  UseCCode=off  RelTol=0.001  AbsTol=1e-06  MinStep=1e-09  ToWorkspace=off  RevertToSquareIcSolve=off  NumHomotopyIterations=100  PhasorMode=off  PhasorModeNumHarmonics=1  DoDC=off  ResidualTolerance=1e-5  UseLocalSolver=off  LocalSolverChoice=NE_TRAPEZOIDAL_ADVANCER  LocalSolverSampleTime=0.00001  DoFixedCost=off  MaxNonlinIter=3  MaxModeIter=2  LinearAlgebra=auto  EquationFormulation=NE_TIME_EF  DelaysMemoryBudget=1024  AutomaticFiltering=on  FilteringTimeConstant=0.0001  PartitionStorageMethod=AS_NEEDED  PartitionMemoryBudget=1024
  World : sm_lib/Frames and Transforms/World Frame
  cetvrti_clanak_1_RIGID : Subsystem
  drugi_clanak_1_RIGID : Subsystem
  hidraulicki_rot_1 : Subsystem
  hidraulicki_trans1_1 : Subsystem
  hidraulicki_trans2_2 : Subsystem
  postolje_1_RIGID : Subsystem
  prvi_clanak_2_RIGID : Subsystem
  treci_clanak_1_RIGID : Subsystem
  FzRot : PMIOPort  Side=Left
  vzRot : PMIOPort  Port=2  Side=Left
  FzTrans1 : PMIOPort  Port=3  Side=Left
  vzTrans1 : PMIOPort  Port=4  Side=Left
  FzTrans2 : PMIOPort  Port=5  Side=Left
  vzTrans2 : PMIOPort  Port=6  Side=Left
  TBase : PMIOPort  Port=7  Side=Left
  wBase : PMIOPort  Port=8  Side=Left
  TPulley : PMIOPort  Port=9  Side=Left
  wPulley : PMIOPort  Port=10  Side=Left
  pzRot : PMIOPort  Port=11  Side=Right
  VzRot : PMIOPort  Port=12  Side=Right
  pzTrans1 : PMIOPort  Port=13  Side=Right
  VzTrans1 : PMIOPort  Port=14  Side=Right
  pzTrans2 : PMIOPort  Port=15  Side=Right
  VzTrans2 : PMIOPort  Port=16  Side=Right
  qBase : PMIOPort  Port=17  Side=Right
  WBase : PMIOPort  Port=18  Side=Right
  qPulley : PMIOPort  Port=19  Side=Right
  WPulley : PMIOPort  Port=20  Side=Right
  xLoad : PMIOPort  Port=21  Side=Right
  yLoad : PMIOPort  Port=22  Side=Right
  zLoad : PMIOPort  Port=23  Side=Right
  vxLoad : PMIOPort  Port=24  Side=Right
  vyLoad : PMIOPort  Port=25  Side=Right
  vzLoad : PMIOPort  Port=26  Side=Right
  xTop : PMIOPort  Port=27  Side=Right
  yTop : PMIOPort  Port=28  Side=Right
  zTop : PMIOPort  Port=29  Side=Right
  vxTop : PMIOPort  Port=30  Side=Right
  vyTop : PMIOPort  Port=31  Side=Right
  vzTop : PMIOPort  Port=32  Side=Right
  connections:
  Cylindrical2/RConn1 -- hidraulicki_trans1_1/LConn4
  MechanismConfiguration/RConn1 -- Solver Configuration/RConn1 -- World/RConn1 -- Rigid Transform1/LConn1 -- Rigid Transform2/LConn1 -- Rigid Transform3/LConn1 -- Rigid Transform/LConn1
  Revolute4/LConn1 -- postolje_1_RIGID/RConn1
  Revolute1/LConn1 -- prvi_clanak_2_RIGID/RConn2
  Revolute2/RConn1 -- hidraulicki_trans2_2/LConn3
  Revolute4/RConn1 -- prvi_clanak_2_RIGID/LConn1
  Cylindrical1/LConn1 -- hidraulicki_rot_1/RConn3
  Parallel/LConn1 -- drugi_clanak_1_RIGID/RConn1
  Revolute3/LConn1 -- prvi_clanak_2_RIGID/RConn1
  Prismatic/LConn1 -- treci_clanak_1_RIGID/RConn3
  Cylindrical1/RConn1 -- drugi_clanak_1_RIGID/LConn1
  Prismatic/RConn1 -- cetvrti_clanak_1_RIGID/LConn1
  Cylindrical2/LConn1 -- treci_clanak_1_RIGID/RConn1
  Revolute/LConn1 -- drugi_clanak_1_RIGID/RConn3
  Parallel/RConn1 -- hidraulicki_trans1_1/LConn3
  Revolute1/RConn1 -- drugi_clanak_1_RIGID/LConn2
  Prismatic1/LConn1 -- drugi_clanak_1_RIGID/RConn2
  Cylindrical/RConn1 -- hidraulicki_trans2_2/LConn4
  Revolute3/RConn1 -- hidraulicki_rot_1/LConn3
  Revolute/RConn1 -- hidraulicki_trans1_1/LConn5
  Prismatic1/RConn1 -- treci_clanak_1_RIGID/LConn1
  Cylindrical/LConn1 -- cetvrti_clanak_1_RIGID/RConn1
  Revolute2/LConn1 -- treci_clanak_1_RIGID/RConn2
  hidraulicki_rot_1/LConn2 -- vzRot/RConn1
  FzRot/RConn1 -- hidraulicki_rot_1/LConn1
  FzTrans1/RConn1 -- hidraulicki_trans1_1/LConn1
  vzTrans1/RConn1 -- hidraulicki_trans1_1/LConn2
  FzTrans2/RConn1 -- hidraulicki_trans2_2/LConn1
  hidraulicki_trans2_2/LConn2 -- vzTrans2/RConn1
  prvi_clanak_2_RIGID/LConn2 -- BeltAndPulley/LConn1
  BeltAndPulley/RConn1 -- cetvrti_clanak_1_RIGID/RConn2
  BeltAndPulley/LConn2 -- TPulley/RConn1
  TBase/RConn1 -- Revolute4/LConn2
  wPulley/RConn1 -- WPulley/RConn1 -- BeltAndPulley/LConn3
  pzRot/RConn1 -- hidraulicki_rot_1/RConn1
  VzRot/RConn1 -- hidraulicki_rot_1/RConn2
  VzTrans1/RConn1 -- hidraulicki_trans1_1/RConn2
  pzTrans1/RConn1 -- hidraulicki_trans1_1/RConn1
  VzTrans2/RConn1 -- hidraulicki_trans2_2/RConn2
  hidraulicki_trans2_2/RConn1 -- pzTrans2/RConn1
  wBase/RConn1 -- Revolute4/RConn3 -- WBase/RConn1
  qBase/RConn1 -- Revolute4/RConn2
  qPulley/RConn1 -- BeltAndPulley/LConn4
  BeltAndPulley/RConn2 -- xLoad/RConn1
  BeltAndPulley/RConn3 -- yLoad/RConn1
  BeltAndPulley/RConn4 -- zLoad/RConn1
  BeltAndPulley/RConn5 -- vxLoad/RConn1
  BeltAndPulley/RConn6 -- vyLoad/RConn1
  BeltAndPulley/RConn7 -- vzLoad/RConn1
  BeltAndPulley/RConn12 -- vyTop/RConn1
  BeltAndPulley/RConn11 -- vxTop/RConn1
  BeltAndPulley/RConn10 -- zTop/RConn1
  BeltAndPulley/RConn8 -- xTop/RConn1
  BeltAndPulley/RConn9 -- yTop/RConn1
  vzTop/RConn1 -- BeltAndPulley/RConn13
  Rigid Transform/RConn1 -- postolje_1_RIGID/LConn1
  Point1/RConn1 -- Rigid Transform1/RConn1
  Point2/RConn1 -- Rigid Transform2/RConn1
  Point3/RConn1 -- Rigid Transform3/RConn1

== system kranTest/Crane/Electromotor Base ==
  Controlled Voltage Source : fl_lib/Electrical/Electrical Sources/Controlled Voltage Source
  DC Motor : elec_lib/Actuators & Drivers/Rotational Actuators/DC Motor  parameterization=1  Ra=3.9 Ohm  La=22e-3 H  emf_or_torque=1  Kv=1.8 V/(rad/s)  Ki=6.876e-4 N*m/A  T_stall=0.24e-3 N*m  w_max=2000 rpm  w_rated=1500 rpm  P_rated=50 kW  V_rated=350 V  J=0.2 kg*m^2  lam_param=1  lam=0 N*m/(rad/s)  i_noload=0 A  V_i_noload=1.5 V  speed0=0 rpm  alpha=3.93e-3 1/K  Tmeas=25 degC  thermal_mass=100 J/K  initial_temperature=25 degC
  Electrical Reference : fl_lib/Electrical/Electrical Elements/Electrical Reference
  Gear Box : fl_lib/Mechanical/Mechanisms/Gear Box  ratio=250  t_in_specify=off  t_in_priority=None  t_in=0 N*m  t_in_nominal_specify=off  t_in_nominal_unit=N*m  t_in_nominal_value=1  t_out_specify=off  t_out_priority=None  t_out=0 N*m  t_out_nominal_specify=off  t_out_nominal_unit=N*m  t_out_nominal_value=1
  Mechanical Rotational Reference : fl_lib/Mechanical/Rotational Elements/Mechanical Rotational Reference
  PS Saturation : fl_lib/Physical Signals/Nonlinear Operators/PS Saturation  upper_limit=250  lower_limit=-250
      settings: SourceProductName=Simscape  SourceProductBaseCode=SS
  Rotation converter : Subsystem
  T : PMIOPort  Side=Right
  w : PMIOPort  Port=2  Side=Right
  voltage : PMIOPort  Port=3  Side=Left
  connections:
  T/RConn1 -- Rotation converter/LConn1
  w/RConn1 -- Rotation converter/RConn1
  DC Motor/RConn2 -- Mechanical Rotational Reference/LConn1 -- Rotation converter/LConn2
  Gear Box/LConn1 -- DC Motor/LConn2
  Gear Box/RConn1 -- Rotation converter/RConn2
  Controlled Voltage Source/LConn1 -- DC Motor/LConn1
  Controlled Voltage Source/RConn2 -- Electrical Reference/LConn1 -- DC Motor/RConn1
  PS Saturation/RConn1 -- Controlled Voltage Source/RConn1
  PS Saturation/LConn1 -- voltage/RConn1

== system kranTest/Crane/Electromotor Pulley ==
  Controlled Voltage Source : fl_lib/Electrical/Electrical Sources/Controlled Voltage Source
  DC Motor : elec_lib/Actuators & Drivers/Rotational Actuators/DC Motor  parameterization=1  Ra=2.7 Ohm  La=12e-3 H  emf_or_torque=1  Kv=1.6 V/(rad/s)  Ki=6.876e-4 N*m/A  T_stall=0.24e-3 N*m  w_max=2000 rpm  w_rated=1500 rpm  P_rated=50 kW  V_rated=350 V  J=0.1 kg*m^2  lam_param=1  lam=0 N*m/(rad/s)  i_noload=0 A  V_i_noload=1.5 V  speed0=0 rpm  alpha=3.93e-3 1/K  Tmeas=25 degC  thermal_mass=100 J/K  initial_temperature=25 degC
  Electrical Reference : fl_lib/Electrical/Electrical Elements/Electrical Reference
  Gear Box : fl_lib/Mechanical/Mechanisms/Gear Box  ratio=20  t_in_specify=off  t_in_priority=None  t_in=0 N*m  t_in_nominal_specify=off  t_in_nominal_unit=N*m  t_in_nominal_value=1  t_out_specify=off  t_out_priority=None  t_out=0 N*m  t_out_nominal_specify=off  t_out_nominal_unit=N*m  t_out_nominal_value=1
  Mechanical Rotational Reference : fl_lib/Mechanical/Rotational Elements/Mechanical Rotational Reference
  PS Saturation : fl_lib/Physical Signals/Nonlinear Operators/PS Saturation  upper_limit=180  lower_limit=-180
      settings: SourceProductName=Simscape  SourceProductBaseCode=SS
  Rotation converter : Subsystem
  T : PMIOPort  Side=Right
  w : PMIOPort  Port=2  Side=Right
  voltage : PMIOPort  Port=3  Side=Left
  connections:
  T/RConn1 -- Rotation converter/LConn1
  w/RConn1 -- Rotation converter/RConn1
  DC Motor/RConn2 -- Mechanical Rotational Reference/LConn1 -- Rotation converter/LConn2
  Controlled Voltage Source/LConn1 -- DC Motor/LConn1
  Controlled Voltage Source/RConn2 -- Electrical Reference/LConn1 -- DC Motor/RConn1
  Gear Box/LConn1 -- DC Motor/LConn2
  Gear Box/RConn1 -- Rotation converter/RConn2
  PS Saturation/RConn1 -- Controlled Voltage Source/RConn1
  PS Saturation/LConn1 -- voltage/RConn1
